simulink model "TR_Single_Coupler"  (Simulink 6.6)
settings: Solver=ode45  StartTime=0.0  StopTime=10.0  RelTol=1e-3
values from neighbouring files (symbols this model uses):
  Bc = 0    [TFconfirm.m]    (also in Torsonal_Model_Constants.m = 0.01)
  Ja = Ja+JL    (= 0.0056)    [TFconfirm.m]
  JL = 0.0033    [TFconfirm.m]    (also in Torsonal_Model_Constants.m)
  Kc = 0    [TFconfirm.m]
settings Model: Creator=Geovana  LastModifiedBy=Geovana

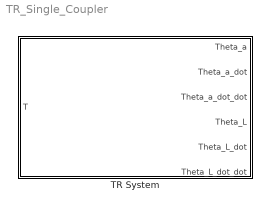
== system TR_Single_Coupler ==
  TR System : Subsystem

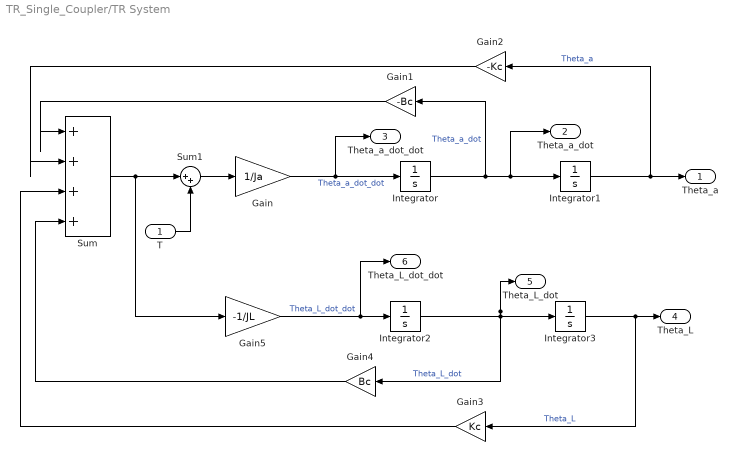
== system TR_Single_Coupler/TR System ==
  T : Inport
  Gain : Gain  Gain=1/Ja
  Gain1 : Gain  Orientation=left  Gain=-Bc
  Gain2 : Gain  Orientation=left  Gain=-Kc
  Gain3 : Gain  Orientation=left  Gain=Kc
  Gain4 : Gain  Orientation=left  Gain=Bc
  Gain5 : Gain  Gain=-1/JL
  Integrator{,1..3} (4 alike) : Integrator
  Sum : Sum  Inputs=|++++
  Sum1 : Sum  Inputs=|++
  Theta_a : Outport
  Theta_a_dot : Outport  Port=2
  Theta_a_dot_dot : Outport  Port=3
  Theta_L : Outport  Port=4
  Theta_L_dot : Outport  Port=5
  Theta_L_dot_dot : Outport  Port=6
  wires:
  Sum/1 -> Gain5/1, Sum1/1
  Integrator/1 -> Gain1/1, Integrator1/1, Theta_a_dot/1  "Theta_a_dot"
  Integrator1/1 -> Gain2/1, Theta_a/1  "Theta_a"
  Gain1/1 -> Sum/1
  Gain2/1 -> Sum/2
  Gain/1 -> Integrator/1, Theta_a_dot_dot/1  "Theta_a_dot_dot"
  Integrator2/1 -> Integrator3/1, Gain4/1, Theta_L_dot/1  "Theta_L_dot"
  Gain5/1 -> Integrator2/1, Theta_L_dot_dot/1  "Theta_L_dot_dot"
  Sum1/1 -> Gain/1
  T/1 -> Sum1/2
  Integrator3/1 -> Theta_L/1, Gain3/1  "Theta_L"
  Gain3/1 -> Sum/3
  Gain4/1 -> Sum/4
